simulink model "Modele_Lineaire"  (R2024a)
settings: Solver=VariableStepAuto  StartTime=0.0  StopTime=1  RelTol=1e-3
undefined symbols (not defined in the file or in its folder): num
settings Model: Creator=francoisdesautels  LastModifiedBy=francoisdesautels

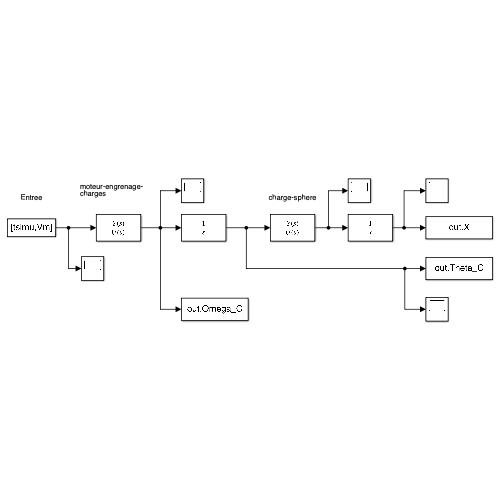
[thumbnail: Simulink's stored preview of the top-level diagram]
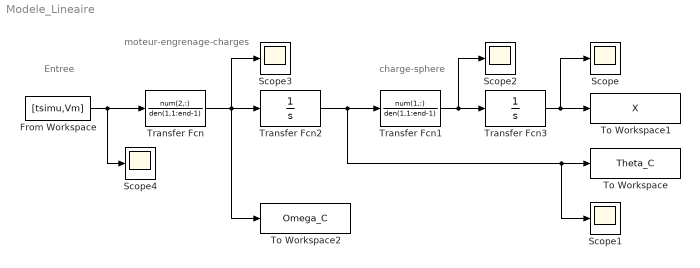
== system Modele_Lineaire ==
  note: charge-sphere
  note: moteur-engrenage-charges
  note: Entree
  From Workspace : FromWorkspace  VariableName=[tsimu,Vm]  SampleTime=-1
  Scope{,1..4} (5 alike) : Scope
  To Workspace : ToWorkspace  VariableName=Theta_C  SaveFormat=Timeseries  SampleTime=-1
      settings: Save2DSignal=2-D array (concatenate along first dimension)
  To Workspace1 : ToWorkspace  VariableName=X  SaveFormat=Timeseries  SampleTime=-1
  To Workspace2 : ToWorkspace  VariableName=Omega_C  SampleTime=-1
  Transfer Fcn : TransferFcn  Numerator=num(2,:)  Denominator=den(1,1:end-1)
  Transfer Fcn1 : TransferFcn  Numerator=num(1,:)  Denominator=den(1,1:end-1)
  Transfer Fcn2 : TransferFcn  Denominator=[1 0]
  Transfer Fcn3 : TransferFcn  Denominator=[1 0]
  wires:
  Transfer Fcn/1 -> To Workspace2/1, Scope3/1, Transfer Fcn2/1
  Transfer Fcn1/1 -> Scope2/1, Transfer Fcn3/1
  Transfer Fcn2/1 -> Transfer Fcn1/1, Scope1/1, To Workspace/1
  Transfer Fcn3/1 -> Scope/1, To Workspace1/1
  From Workspace/1 -> Scope4/1, Transfer Fcn/1
